simulink model "kof_halozat"  (R2020a)
settings: Solver=VariableStepAuto  StartTime=0.0  StopTime=10.0  RelTol=1e-3
undefined symbols (not defined in the file): D1, Delta
libraries: powerlib x5, factslib x1
settings Model: Creator=Ákos  LastModifiedBy=Ákos

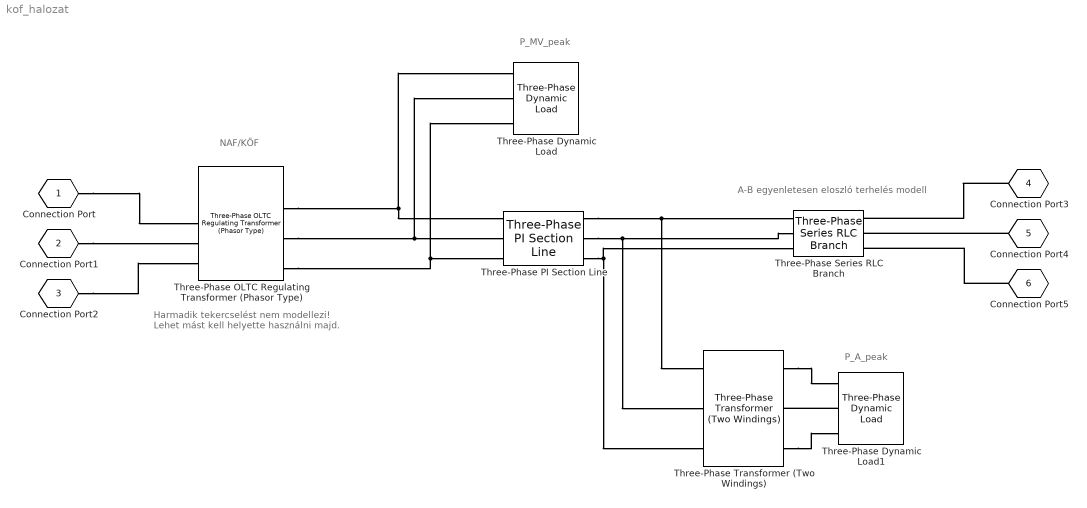
== system kof_halozat ==
  note: A-B egyenletesen eloszló terhelés modell
  note: P_MV_peak
  note: NAF/KÖF
  note: Harmadik tekercselést
      | nem modellezi!
      |
      | Lehet mást kell helyette használni majd.
  note: P_A_peak
  Three-Phase Dynamic Load : powerlib/Elements/Three-Phase Dynamic Load  NominalVoltage=[ 500e3 60 ]  ActiveReactivePowers=[50e6 25e6]  PositiveSequence=[0.994 -11.8]  ExternalControl=off  NpNq=[1.3 2]  TimeConstants="[0  0  0  0]"  MinimumVoltage=0.7  Tfilter=1e-4  LoadFlowParameters=[4,0,0,0,0]
      settings: SourceProductBaseCode=PS
  Three-Phase Dynamic Load1 : powerlib/Elements/Three-Phase Dynamic Load  NominalVoltage=[ 500e3 60 ]  ActiveReactivePowers=[50e6 25e6]  PositiveSequence=[0.994 -11.8]  ExternalControl=off  NpNq=[1.3 2]  TimeConstants="[0  0  0  0]"  MinimumVoltage=0.7  Tfilter=1e-4  LoadFlowParameters=[4,0,0,0,0]
      settings: SourceProductBaseCode=PS
  Three-Phase PI Section Line : powerlib/Elements/Three-Phase PI Section Line  LConnTagsString=a|b|c  RConnTagsString=A|B|C  Frequency=50  Resistances=[ 0.01273 0.3864]  Inductances="[ 0.9337e-3  4.1264e-3]"  Capacitances=[12.74e-9 7.751e-9]  Length=1
  Three-Phase Series RLC Branch : powerlib/Elements/Three-Phase Series RLC Branch  LConnTagsString=A|B|C  RConnTagsString=A|B|C  BranchType=RLC  Resistance=1  Inductance=1e-3  Capacitance=1e-6  Measurements=None
  Three-Phase Transformer (Two Windings) : powerlib/Elements/Three-Phase Transformer (Two Windings)  Winding1Connection=Delta (D1)  Winding2Connection=Y  CoreType=Three single-phase transformers  SetSaturation=off  Hysteresis=off  DataFile='hysteresis'  SetInitialFlux=off  Measurements=None  UNITS=pu  NominalPower=[ 250e6 , 60 ]  Winding1=[ 735e3 , 0.002 , 0.08 ]  Winding2=[ 315e3 , 0.002 , 0.08 ]  Rm=500  Lm=500  L0=0.5  Saturation=[ 0,0 ; 0.0024,1.2 ; 1.0,1.52 ]  InitialFluxes=[ 0.8 , -0.8 , 0.7 ]  BreakLoop=off  DiscreteSolver=Trapezoidal iterative  DataType=off  TransfoNumber=1
  Three-Phase OLTC Regulating Transformer (Phasor Type) : factslib/Transformers/Three-Phase OLTC Regulating Transformer (Phasor Type)  Winding1Connection=Y  Winding2Connection=Y  PnomFnom="[47e6,  60]"  Winding1=[120e3, 0.003, 0.09 ]  Winding2="[25e3,  0.003, 0.09 ]"  Iw2_init=[0.7568, -45]  RmXm=[300, 300]  TapOnWinding=Winding 1  WindingTap=[ 0.003, 0.09]  dU=0.01875  TapMinMax=[ -8, +8]  InitialTap=-4  TapSelectionTime=4  ExternalControl=on  RegulatorOn=on  Regulator="[1.04,  0.0375, 1]"
      settings: SourceProductBaseCode=PS
  Connection Port : PMIOPort  Tag=PMCPort  Side=Left
  Connection Port1 : PMIOPort  Tag=PMCPort  Port=2  Side=Left
  Connection Port2 : PMIOPort  Tag=PMCPort  Port=3  Side=Left
  Connection Port3 : PMIOPort  Tag=PMCPort  Port=4  Side=Left
  Connection Port4 : PMIOPort  Tag=PMCPort  Port=5  Side=Left
  Connection Port5 : PMIOPort  Tag=PMCPort  Port=6  Side=Left
  connections:
  Three-Phase OLTC Regulating Transformer (Phasor Type)/RConn1 -- Three-Phase PI Section Line/LConn1 -- Three-Phase Dynamic Load/LConn1
  Three-Phase OLTC Regulating Transformer (Phasor Type)/RConn2 -- Three-Phase PI Section Line/LConn2 -- Three-Phase Dynamic Load/LConn2
  Three-Phase OLTC Regulating Transformer (Phasor Type)/RConn3 -- Three-Phase PI Section Line/LConn3 -- Three-Phase Dynamic Load/LConn3
  Three-Phase PI Section Line/RConn1 -- Three-Phase Series RLC Branch/LConn1 -- Three-Phase Transformer (Two Windings)/LConn1
  Three-Phase PI Section Line/RConn2 -- Three-Phase Series RLC Branch/LConn2 -- Three-Phase Transformer (Two Windings)/LConn2
  Three-Phase PI Section Line/RConn3 -- Three-Phase Series RLC Branch/LConn3 -- Three-Phase Transformer (Two Windings)/LConn3
  Three-Phase Dynamic Load1/LConn2 -- Three-Phase Transformer (Two Windings)/RConn2
  Three-Phase Transformer (Two Windings)/RConn1 -- Three-Phase Dynamic Load1/LConn1
  Three-Phase Transformer (Two Windings)/RConn3 -- Three-Phase Dynamic Load1/LConn3
  Connection Port/RConn1 -- Three-Phase OLTC Regulating Transformer (Phasor Type)/LConn1
  Connection Port1/RConn1 -- Three-Phase OLTC Regulating Transformer (Phasor Type)/LConn2
  Connection Port2/RConn1 -- Three-Phase OLTC Regulating Transformer (Phasor Type)/LConn3
  Connection Port4/RConn1 -- Three-Phase Series RLC Branch/RConn2
  Connection Port3/RConn1 -- Three-Phase Series RLC Branch/RConn1
  Connection Port5/RConn1 -- Three-Phase Series RLC Branch/RConn3
